simulink model "Continuos_plant_LTV_system"  (R2016b)
settings: Solver=ode3  StartTime=0.0  StopTime=1  FixedStep=0.01  RelTol=1e-6
libraries: dspinverses x1
settings Model: Creator=Utente  LastModifiedBy=liana
settings DataIOCC: SaveState=on
settings OptimizationCC: BlockReduction=off  DefaultParameterBehavior=Inlined  BufferReuse=off

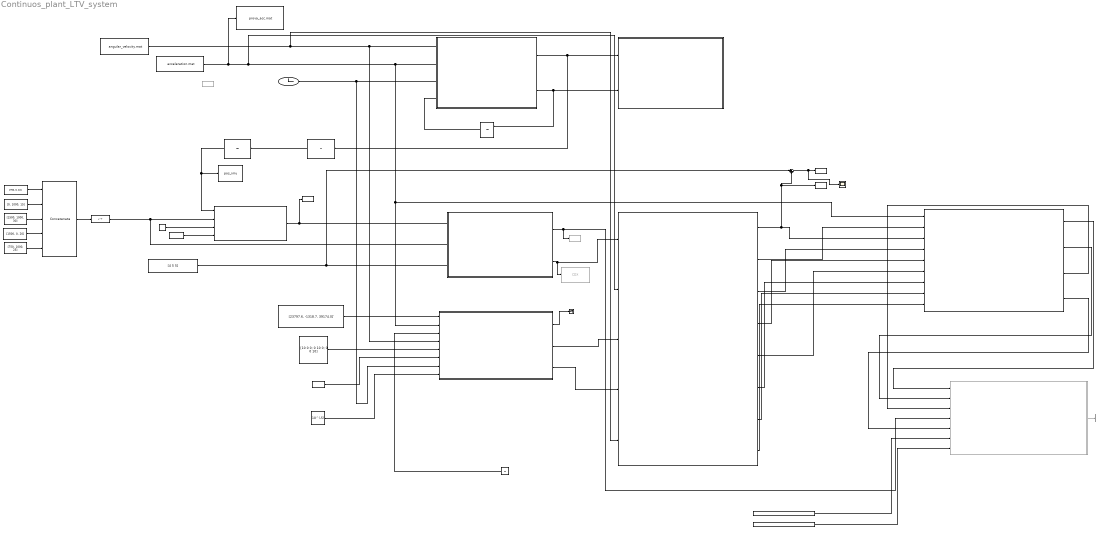
== system Continuos_plant_LTV_system ==
  Attitude Observer : Subsystem
  Clock : Clock
      settings: Decimation=50
  Displays : Subsystem
  From acceleration file : FromFile  FileName=acceleration.mat  SampleTime=0
  From angular_velocity file : FromFile  FileName=angular_velocity.mat  SampleTime=0
  Integrator : Integrator  InitialConditionSource=external
  Integrator1 : Integrator
  Integrator2 : Integrator
  Kalman - Bucy Filter : Subsystem  Commented=on
  Kp : Constant  Value=[10 0 0; 0 10 0; 0 0 10]
  Local linearization1 : Subsystem
  Math Function : Math  Operator=transpose  SaturateOnIntegerOverflow=on
  Matrix Concatenate (transponders positions) : Concatenate  NumInputs=5  Mode=Multidimensional array  ConcatenateDimension=2
  Mechanisation subsystem : Subsystem
  Nonlinear algebraic transform and solution : Subsystem
  Q matrix : Constant  Value=diag([0, 0, 0, 10^-5, 10^-3, 10^-3, 10^-3, 10^-8, 10^-8, 10^-8])
  R matrix : Constant  Value=0.25*diag([1 1 1 1])
  Scope : Scope
  Sum : Sum  Inputs=|++
  Terminator1 : Terminator
  Terminator2 : Terminator  Commented=on
  To File : ToFile  Filename=prova_acc.mat  MatrixName=prova_acc  SaveFormat=Timeseries
  To Workspace : ToWorkspace  VariableName=pseudo  SaveFormat=Timeseries  SampleTime=-1
  To Workspace1 : ToWorkspace  VariableName=pos_imu  SaveFormat=Timeseries  SampleTime=-1
  To Workspace2 : ToWorkspace  Commented=on  VariableName=CDX  SaveFormat=Timeseries  SampleTime=-1
  To Workspace3 : ToWorkspace  Commented=on  VariableName=acc_test  SaveFormat=Timeseries  SampleTime=-1
  To Workspace4 : ToWorkspace  VariableName=p_n  SaveFormat=Timeseries  SampleTime=-1
  To Workspace5 : ToWorkspace  VariableName=p_n_delta_stim  SaveFormat=Timeseries  SampleTime=-1
  To Workspace6 : ToWorkspace  Commented=on  VariableName=delta  SaveFormat=Timeseries  SampleTime=-1
  Translational Motion Observer : Subsystem
  Unit Delay : UnitDelay  SampleTime=-1
  beta : Constant
  epsilon : Constant  Value=[1 1 1 1 1]*0.1
  ki : Constant  Value=10^(-5)
  magneto_values (Pisa) : Constant  Value=[23797.6, -1318.7, 39174.0]'
  p_n_1 : Constant  Value=[750, 0, 10]
  p_n_2 : Constant  Value=[0, 1000, 15]
  p_n_3 : Constant  Value=[1500, 1000, 30]
  p_n_4 : Constant  Value=[1500, 0, 20]
  p_n_5 : Constant  Value=[750, 1000, 25]
  position_0_fixed_reference : Constant  Value=[4 5 5]
  pseudorange_measurement_model : MATLAB Function  TreatAsAtomicUnit=on
  sigma : Constant  Value=0.25
  wires:
  Clock/1 -> Attitude Observer/7(t), Mechanisation subsystem/3(t)
  Mechanisation subsystem/1(v_n_dot) -> Integrator1/1, Displays/1(v_n_dot)
  Mechanisation subsystem/2(R_nb_dot) -> Integrator/1, Displays/2(R_nb_dot)
  Nonlinear algebraic transform and solution/1(delta) -> To Workspace6/1, Kalman - Bucy Filter/4(sensors measurements)
  Kp/1 -> Attitude Observer/5(Kp)
  sigma/1 -> Attitude Observer/6(sigma)
  Nonlinear algebraic transform and solution/2(C_dx) -> Translational Motion Observer/1(C_dx_), To Workspace2/1
  Local linearization1/1(AL) -> Kalman - Bucy Filter/1(AL)
  Local linearization1/2(BL) -> Kalman - Bucy Filter/2(BL)
  Local linearization1/3(CL) -> Kalman - Bucy Filter/3(CL)
  pseudorange_measurement_model/1(y) -> To Workspace/1, Nonlinear algebraic transform and solution/1(y)
  Local linearization1/4(U) -> Kalman - Bucy Filter/5(U)
  beta/1 -> pseudorange_measurement_model/3(beta)
  epsilon/1 -> pseudorange_measurement_model/4(epsilon)
  Matrix Concatenate (transponders positions)/1 -> Math Function/1
  R matrix/1 -> Kalman - Bucy Filter/6(R)
  Q matrix/1 -> Kalman - Bucy Filter/7(Q)
  Kalman - Bucy Filter/1(Out1) -> Terminator2/1
  ki/1 -> Attitude Observer/8(Ki)
  Unit Delay/1 -> Attitude Observer/3(f_n_stim)
  p_n_5/1 -> Matrix Concatenate (transponders positions)/5
  p_n_4/1 -> Matrix Concatenate (transponders positions)/4
  p_n_3/1 -> Matrix Concatenate (transponders positions)/3
  p_n_2/1 -> Matrix Concatenate (transponders positions)/2
  p_n_1/1 -> Matrix Concatenate (transponders positions)/1
  Math Function/1 -> Nonlinear algebraic transform and solution/2(p), pseudorange_measurement_model/2(p_n_i)
  From angular_velocity file/1 -> Translational Motion Observer/5(w_b_ib_), Attitude Observer/4(w_ib), Mechanisation subsystem/1(w_ib)
  From acceleration file/1 -> To File/1, Translational Motion Observer/2(f_b_), Local linearization1/1(f_b_imu), Attitude Observer/2(f_b), Mechanisation subsystem/2(f_b)
  Sum/1 -> Scope/1, To Workspace4/1
  position_0_fixed_reference/1 -> Sum/1, Nonlinear algebraic transform and solution/3(p0)
  Integrator/1 -> Mechanisation subsystem/4("R_nb ")
  Integrator2/1 -> To Workspace1/1, pseudorange_measurement_model/1(p_n)
  magneto_values (Pisa)/1 -> Attitude Observer/1(m_b_mag)
  Integrator1/1 -> Integrator2/1
  Translational Motion Observer/2(beta_stim_) -> Local linearization1/2(beta_stim)
  Translational Motion Observer/5(K_) -> Local linearization1/6(K)
  Translational Motion Observer/1(p_n_delta_stim_) -> Sum/2, To Workspace5/1, Local linearization1/3(p_n_delta_stim)
  Translational Motion Observer/3(v_n_stim_) -> Local linearization1/4(v_n_stim)
  Translational Motion Observer/4(f_n_stim_) -> Local linearization1/5(f_n_stim)
  Translational Motion Observer/6(C_) -> Local linearization1/7(C)
  Translational Motion Observer/7(A_) -> Local linearization1/8(A)
  Translational Motion Observer/8(B_1_) -> Local linearization1/9(B)
  Attitude Observer/2(R_nb_stim) -> Translational Motion Observer/3("R_nb_stim_ ")
  Attitude Observer/1(J) -> Terminator1/1
  Attitude Observer/3(b_stim) -> Translational Motion Observer/4(b_stim)

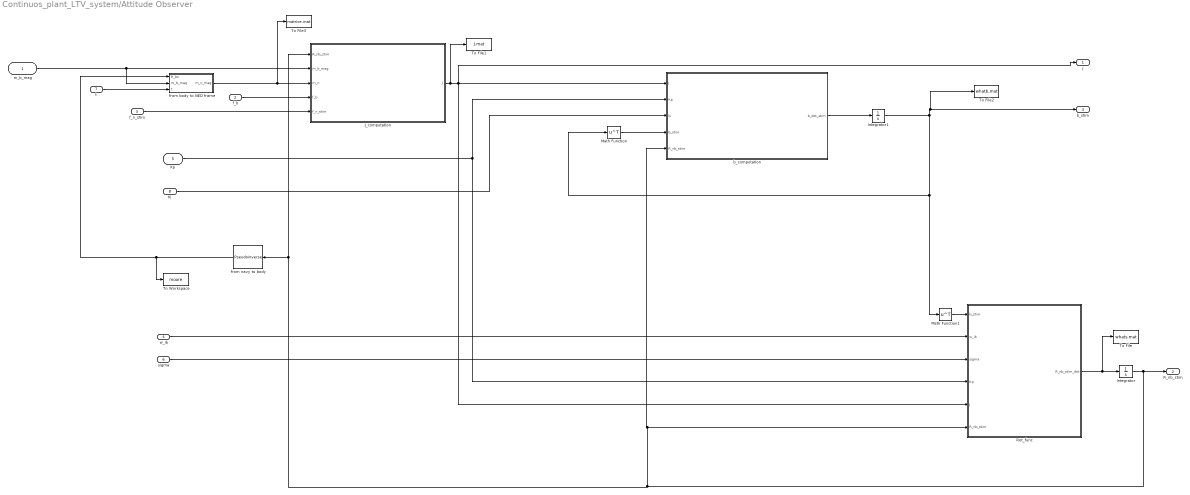
== system Continuos_plant_LTV_system/Attitude Observer ==
  m_b_mag : Inport
  f_b : Inport  Port=2
  f_n_stim : Inport  Port=3
  w_ib : Inport  Port=4
  Kp : Inport  Port=5
  sigma : Inport  Port=6
  t : Inport  Port=7
  Ki : Inport  Port=8
  Integrator : Integrator
  Integrator1 : Integrator
  J_computation : Subsystem
  Math Function : Math  Operator=transpose  SaturateOnIntegerOverflow=on
  Math Function1 : Math  Operator=transpose  SaturateOnIntegerOverflow=on
  Rot_func : MATLAB Function  TreatAsAtomicUnit=on
  To File : ToFile  Filename=whats.mat  MatrixName=ansm  SaveFormat=Timeseries
  To File1 : ToFile  Filename=J.mat  MatrixName=J  SaveFormat=Timeseries
  To File2 : ToFile  Filename=whatb.mat  MatrixName=b  SaveFormat=Timeseries
  To File3 : ToFile  Filename=matrice.mat  MatrixName=m  SaveFormat=Timeseries
  To Workspace : ToWorkspace  VariableName=moore  SaveFormat=Timeseries  SampleTime=-1
  b_computation : MATLAB Function  TreatAsAtomicUnit=on
  from body to NED frame : MATLAB Function  TreatAsAtomicUnit=on
  from navy to body : dspinverses/Pseudoinverse  wanterr=off  SimulateUsing=Interpreted execution
  J : Outport
  R_nb_stim : Outport  Port=2
  b_stim : Outport  Port=3
  wires:
  m_b_mag/1 -> from body to NED frame/2(m_b_mag), J_computation/2(m_b_mag)
  Rot_func/1(R_nb_stim_dot) -> Integrator/1, To File/1
  b_computation/1(b_dot_stim) -> Integrator1/1
  from body to NED frame/1(m_n_mag) -> To File3/1, J_computation/3(m_n)
  f_b/1 -> J_computation/4(f_b)
  f_n_stim/1 -> J_computation/5(f_n_stim)
  J_computation/1(J) -> To File1/1, J/1, Rot_func/5(J), b_computation/1(J)
  Kp/1 -> b_computation/2(Kp), Rot_func/4(Kp)
  Ki/1 -> b_computation/3(ki)
  sigma/1 -> Rot_func/3(sigma)
  w_ib/1 -> Rot_func/2(w_ib)
  t/1 -> from body to NED frame/3(t)
  Integrator1/1 -> Math Function/1, Math Function1/1, To File2/1, b_stim/1
  Integrator/1 -> from navy to body/1, J_computation/1(R_nb_stim), b_computation/5(R_nb_stim), Rot_func/6(R_nb_stim), R_nb_stim/1
  from navy to body/1 -> To Workspace/1, from body to NED frame/1(R_bn)
  Math Function/1 -> b_computation/4(b_stim)
  Math Function1/1 -> Rot_func/1(b_stim)

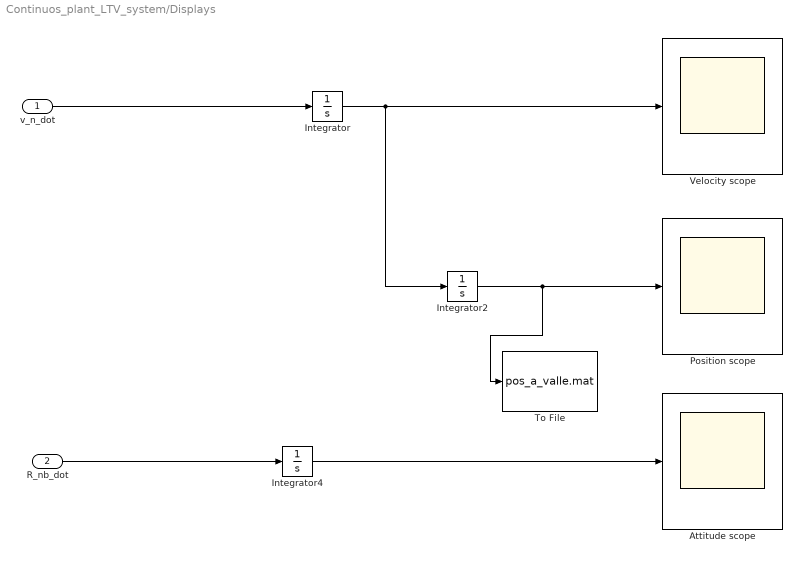
== system Continuos_plant_LTV_system/Displays ==
  v_n_dot : Inport
  R_nb_dot : Inport  Port=2
  Attitude scope : Scope
  Integrator : Integrator
  Integrator2 : Integrator
  Integrator4 : Integrator
  Position scope : Scope
  To File : ToFile  Filename=pos_a_valle.mat  MatrixName=pos_valle  SaveFormat=Timeseries
  Velocity scope : Scope
  wires:
  v_n_dot/1 -> Integrator/1
  Integrator/1 -> Integrator2/1, Velocity scope/1
  Integrator2/1 -> To File/1, Position scope/1
  R_nb_dot/1 -> Integrator4/1
  Integrator4/1 -> Attitude scope/1

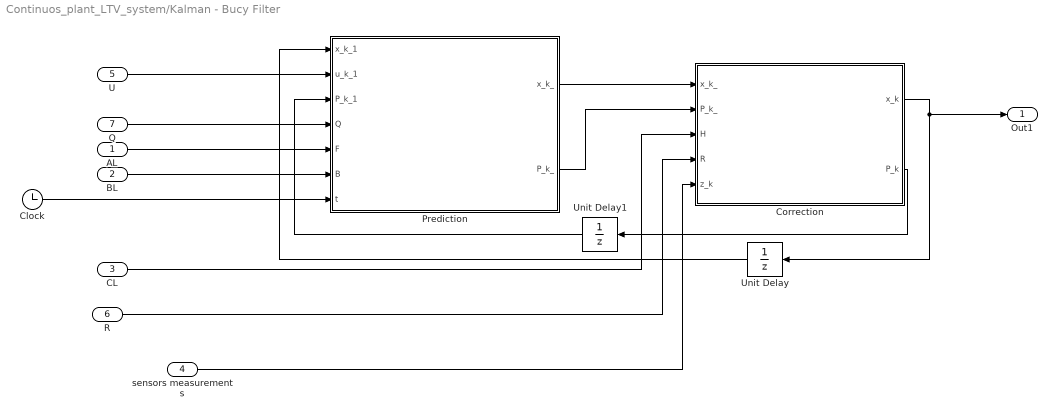
== system Continuos_plant_LTV_system/Kalman - Bucy Filter ==
  AL : Inport
  BL : Inport  Port=2
  CL : Inport  Port=3
  sensors measurements : Inport  Port=4
  U : Inport  Port=5
  R : Inport  Port=6
  Q : Inport  Port=7
  Clock : Clock
  Correction : MATLAB Function  TreatAsAtomicUnit=on
  Prediction : MATLAB Function  TreatAsAtomicUnit=on
  Unit Delay : UnitDelay  SampleTime=-1
  Unit Delay1 : UnitDelay  SampleTime=-1
  Out1 : Outport
  wires:
  Prediction/2(P_k_) -> Correction/2(P_k_)
  Prediction/1(x_k_) -> Correction/1(x_k_)
  Correction/2(P_k) -> Unit Delay1/1
  Correction/1(x_k) -> Unit Delay/1, Out1/1
  AL/1 -> Prediction/5(F)
  CL/1 -> Correction/3(H)
  Clock/1 -> Prediction/7(t)
  Q/1 -> Prediction/4(Q)
  sensors measurements/1 -> Correction/5(z_k)
  BL/1 -> Prediction/6(B)
  U/1 -> Prediction/2(u_k_1)
  R/1 -> Correction/4(R)
  Unit Delay/1 -> Prediction/1(x_k_1)
  Unit Delay1/1 -> Prediction/3(P_k_1)

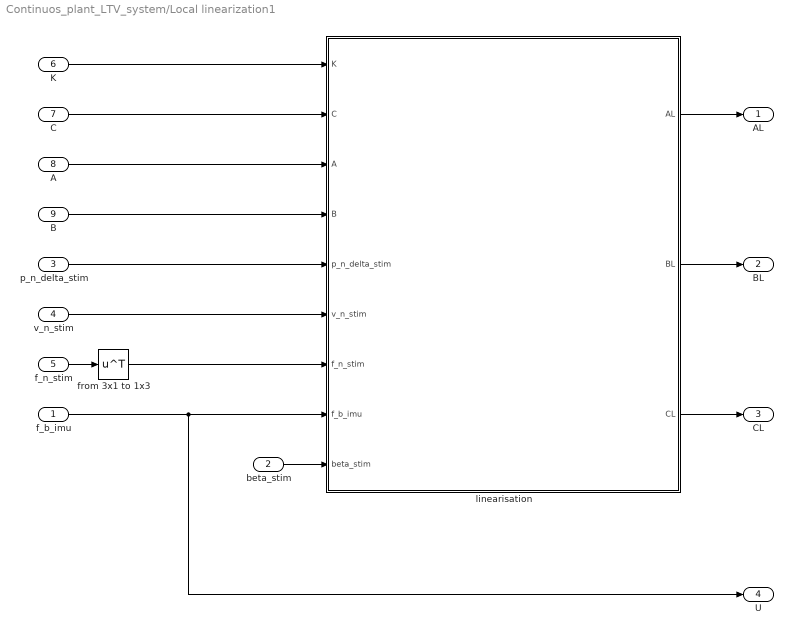
== system Continuos_plant_LTV_system/Local linearization1 ==
  f_b_imu : Inport
  beta_stim : Inport  Port=2
  p_n_delta_stim : Inport  Port=3
  v_n_stim : Inport  Port=4
  f_n_stim : Inport  Port=5
  K : Inport  Port=6
  C : Inport  Port=7
  A : Inport  Port=8
  B : Inport  Port=9
  from 3x1 to 1x3 : Math  Operator=transpose  SaturateOnIntegerOverflow=on
  linearisation : MATLAB Function  TreatAsAtomicUnit=on
  AL : Outport
  BL : Outport  Port=2
  CL : Outport  Port=3
  U : Outport  Port=4
  wires:
  linearisation/1(AL) -> AL/1
  linearisation/2(BL) -> BL/1
  linearisation/3(CL) -> CL/1
  K/1 -> linearisation/1(K)
  C/1 -> linearisation/2(C)
  A/1 -> linearisation/3(A)
  B/1 -> linearisation/4(B)
  p_n_delta_stim/1 -> linearisation/5(p_n_delta_stim)
  beta_stim/1 -> linearisation/9(beta_stim)
  f_n_stim/1 -> from 3x1 to 1x3/1
  v_n_stim/1 -> linearisation/6(v_n_stim)
  from 3x1 to 1x3/1 -> linearisation/7(f_n_stim)
  f_b_imu/1 -> U/1, linearisation/8(f_b_imu)

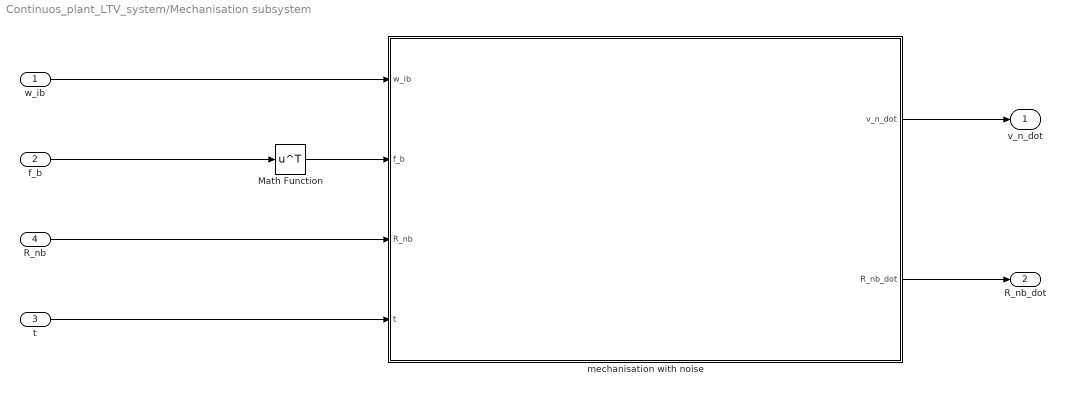
== system Continuos_plant_LTV_system/Mechanisation subsystem ==
  w_ib : Inport
  f_b : Inport  Port=2
  t : Inport  Port=3
  "R_nb " : Inport  Port=4
  Math Function : Math  Operator=transpose  SaturateOnIntegerOverflow=on
  mechanisation with noise : MATLAB Function  TreatAsAtomicUnit=on
  v_n_dot : Outport
  R_nb_dot : Outport  Port=2
  wires:
  w_ib/1 -> mechanisation with noise/1(w_ib)
  t/1 -> mechanisation with noise/4(t)
  f_b/1 -> Math Function/1
  mechanisation with noise/1(v_n_dot) -> v_n_dot/1
  mechanisation with noise/2(R_nb_dot) -> R_nb_dot/1
  "R_nb "/1 -> mechanisation with noise/3(R_nb)
  Math Function/1 -> mechanisation with noise/2(f_b)

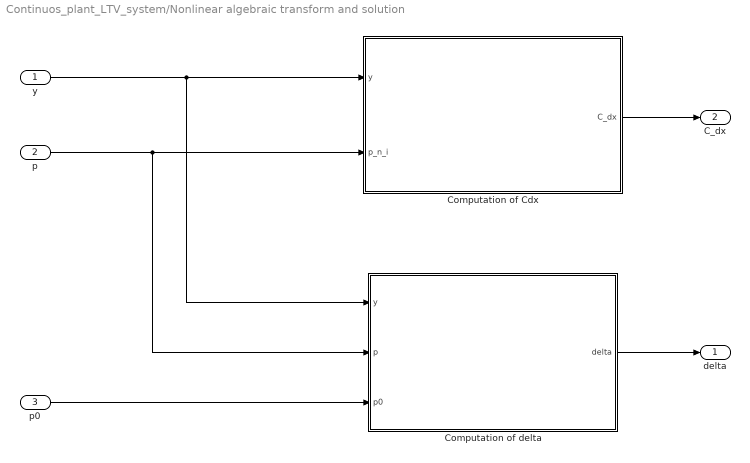
== system Continuos_plant_LTV_system/Nonlinear algebraic transform and solution ==
  y : Inport
  p : Inport  Port=2
  p0 : Inport  Port=3
  Computation of Cdx : MATLAB Function  TreatAsAtomicUnit=on
  Computation of delta : MATLAB Function  TreatAsAtomicUnit=on
  delta : Outport
  C_dx : Outport  Port=2
  wires:
  y/1 -> Computation of delta/1(y), Computation of Cdx/1(y)
  p/1 -> Computation of delta/2(p), Computation of Cdx/2(p_n_i)
  p0/1 -> Computation of delta/3(p0)
  Computation of delta/1(delta) -> delta/1
  Computation of Cdx/1(C_dx) -> C_dx/1

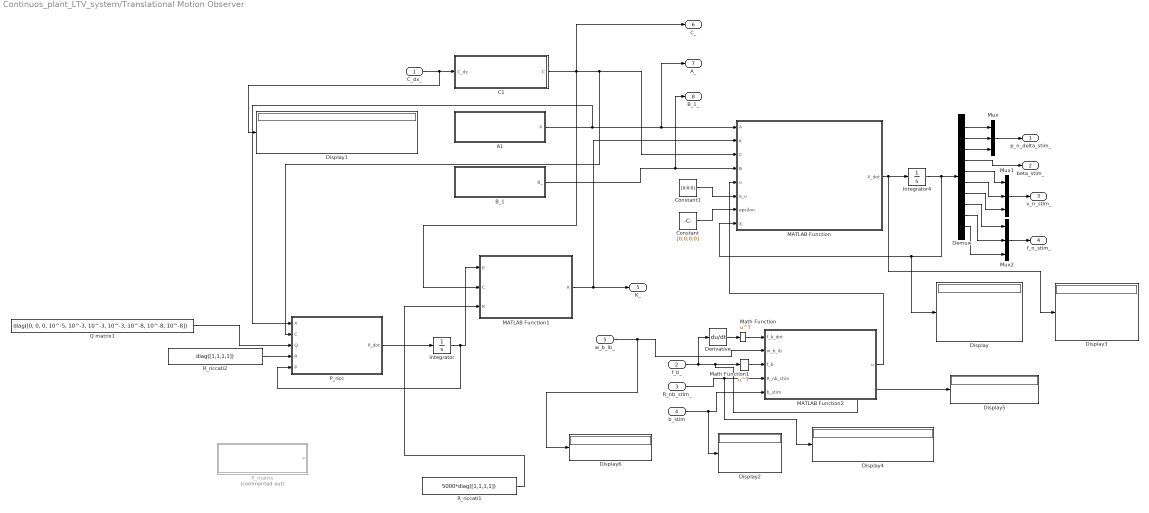
== system Continuos_plant_LTV_system/Translational Motion Observer ==
  C_dx_ : Inport
  f_b_ : Inport  Port=2
  "R_nb_stim_ " : Inport  Port=3
  b_stim : Inport  Port=4
  w_b_ib_ : Inport  Port=5
  A1 : MATLAB Function  TreatAsAtomicUnit=on
  B_1 : MATLAB Function  TreatAsAtomicUnit=on
  C1 : MATLAB Function  TreatAsAtomicUnit=on
  Constant : Constant  Value=[0;0;0;0]
  Constant1 : Constant  Value=[0;0;0]
  Demux : Demux  Outputs=10
  Derivative : Derivative
  Display{,1..6} (7 alike) : Display
  Integrator : Integrator
  Integrator4 : Integrator  AbsoluteTolerance=10^-9
  MATLAB Function : MATLAB Function  TreatAsAtomicUnit=on
  MATLAB Function1 : MATLAB Function  TreatAsAtomicUnit=on
  MATLAB Function2 : MATLAB Function  TreatAsAtomicUnit=on
  Math Function : Math  Operator=transpose  SaturateOnIntegerOverflow=on
  Math Function1 : Math  Operator=transpose  SaturateOnIntegerOverflow=on
  Mux : Mux  Inputs=3
  Mux1 : Mux  Inputs=3
  Mux2 : Mux  Inputs=3
  "P_matrix " : MATLAB Function  Commented=on  TreatAsAtomicUnit=on
  P_ricc : MATLAB Function  TreatAsAtomicUnit=on
  Q matrix1 : Constant  Value=diag([0, 0, 0, 10^-5, 10^-3, 10^-3, 10^-3, 10^-8, 10^-8, 10^-8])
  R_riccati1 : Constant  Value=5000*diag([1,1,1,1])
  R_riccati2 : Constant  Value=diag([1,1,1,1])
  p_n_delta_stim_ : Outport
  beta_stim_ : Outport  Port=2
  v_n_stim_ : Outport  Port=3
  f_n_stim_ : Outport  Port=4
  K_ : Outport  Port=5
  C_ : Outport  Port=6
  A_ : Outport  Port=7
  B_1_ : Outport  Port=8
  wires:
  MATLAB Function/1(X_dot) -> Display3/1, Integrator4/1
  Integrator4/1 -> Demux/1, Display/1, MATLAB Function/8(X)
  Demux/1 -> Mux/1
  Demux/2 -> Mux/2
  Demux/3 -> Mux/3
  Mux/1 -> p_n_delta_stim_/1
  Demux/4 -> beta_stim_/1
  Demux/5 -> Mux1/1
  Demux/6 -> Mux1/2
  Demux/7 -> Mux1/3
  Mux1/1 -> v_n_stim_/1
  Demux/8 -> Mux2/1
  Demux/9 -> Mux2/2
  Demux/10 -> Mux2/3
  Mux2/1 -> f_n_stim_/1
  A1/1(A) -> P_ricc/1(A), A_/1, MATLAB Function/1(A)
  C1/1(C) -> C_/1, MATLAB Function1/2(C), P_ricc/2(C), MATLAB Function/3(C)
  B_1/1(B_) -> B_1_/1, MATLAB Function/4(B)
  C_dx_/1 -> Display1/1, C1/1(C_dx)
  MATLAB Function1/1(K) -> K_/1, MATLAB Function/2(K)
  R_riccati1/1 -> MATLAB Function1/3(R)
  Constant/1 -> MATLAB Function/7(epsilon)
  MATLAB Function2/1(u) -> MATLAB Function/5(u)
  f_b_/1 -> Derivative/1, Display5/1, Math Function1/1
  "R_nb_stim_ "/1 -> Display4/1, MATLAB Function2/4(R_nb_stim)
  b_stim/1 -> Display2/1, MATLAB Function2/5(b_stim)
  w_b_ib_/1 -> Display6/1, MATLAB Function2/2(w_b_ib)
  Constant1/1 -> MATLAB Function/6(e_u)
  P_ricc/1(P_dot) -> Integrator/1
  Integrator/1 -> P_ricc/5(P), MATLAB Function1/1(P)
  R_riccati2/1 -> P_ricc/4(R)
  Q matrix1/1 -> P_ricc/3(Q)
  Derivative/1 -> Math Function/1
  Math Function/1 -> MATLAB Function2/1(f_b_dot)
  Math Function1/1 -> MATLAB Function2/3(f_b)

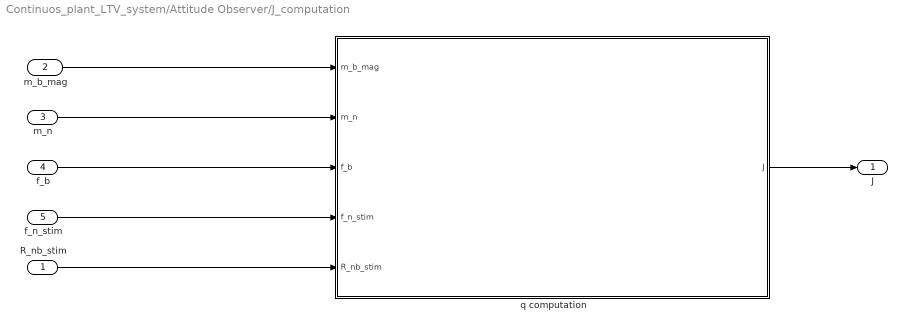
== system Continuos_plant_LTV_system/Attitude Observer/J_computation ==
  R_nb_stim : Inport
  m_b_mag : Inport  Port=2
  m_n : Inport  Port=3
  f_b : Inport  Port=4
  f_n_stim : Inport  Port=5
  q computation : MATLAB Function  TreatAsAtomicUnit=on
  J : Outport
  wires:
  m_n/1 -> q computation/2(m_n)
  f_n_stim/1 -> q computation/4(f_n_stim)
  m_b_mag/1 -> q computation/1(m_b_mag)
  f_b/1 -> q computation/3(f_b)
  q computation/1(J) -> J/1
  R_nb_stim/1 -> q computation/5(R_nb_stim)

== matlab function Continuos_plant_LTV_system/Translational Motion Observer/P_ricc ==
  data: P_dot output size=[10,10]; A input; C input; Q input; R input; P input
function P_dot = P(A, C, Q, R, P)

    P_dot = P*A + A'*P - P*C'*inv(R)*C*P + Q;
 
end

== matlab function Continuos_plant_LTV_system/Attitude Observer/J_computation/q computation ==
  data: m_b_mag input; m_n input; f_b input; f_n_stim input size=3; J output; R_nb_stim input size=[3,3]
function J  = qEfunc(m_b_mag, m_n, f_b, f_n_stim, R_nb_stim)

g_n = [0 0 9.81]';

q1_b = m_b_mag/norm(m_b_mag,2);
q2_b = f_b/norm(g_n,2);

q1_n = m_n/norm(m_n,2);
q2_n = f_n_stim/norm(g_n,2);


E_b = [q1_b, skew(q1_b)*q2_b', (skew(q1_b)*skew(q1_b))*q2_b'];
E_n = [q1_n, skew(q1_n)*q2_n, (skew(q1_n)*skew(q1_n))*q2_n];

J = (E_n - R_nb_stim * E_b) * (E_b');

end

== matlab function Continuos_plant_LTV_system/Kalman - Bucy Filter/Prediction ==
  data: x_k_1 input size=[10, 1]; x_k_ output; u_k_1 input; P_k_1 input size=[10,10]; Q input; F input; B input; P_k_ output; t input
function [x_k_, P_k_] = prediction(x_k_1, u_k_1, P_k_1, Q, F,B, t)

    % initial value of x_k_1
    if t == 0
        x_k_1 = zeros(10,1);
    end

    x_k_ = F * x_k_1 + B * u_k_1';
    
    P_k_ = F * P_k_1 * F' + Q;
    

end

== matlab function Continuos_plant_LTV_system/Mechanisation subsystem/mechanisation with noise ==
  data: w_ib input; f_b input; v_n_dot output; R_nb_dot output; R_nb input; t input
function [v_n_dot, R_nb_dot] = mechanisation(w_ib, f_b, R_nb, t)



g_n = [0 0 1]';

% w_ib = size(3,1);

if t == 0
    v_n_dot = zeros(3,1);
    R_nb_dot = eye(3);
    R_nb = eye(3);
end

Skew = skew(w_ib);


%p_dot = v_n;

v_n_dot = R_nb * f_b + g_n;

R_nb_dot = R_nb * Skew;

== matlab function Continuos_plant_LTV_system/Attitude Observer/b_computation ==
  data: J input; b_dot_stim output size=3; Kp input; ki input; b_stim input; R_nb_stim input
function b_dot_stim = b_dot_stim_func(J, Kp, ki, b_stim, R_nb_stim)

% don't break balls if there are too rows

%b_dot_stim = zeros(3 ,1);

% if t == 0
%    
%     b_stim = zeros(3, 1);
%     
% end

SAT = sat(R_nb_stim)';
PA = pa( SAT * Kp * J);
VEX = vexfunc(PA);
b_dot_stim = Proj(b_stim , -ki * VEX);

end

== matlab function Continuos_plant_LTV_system/Nonlinear algebraic transform and solution/Computation of Cdx ==
  data: y input; p_n_i input; C_dx output size=[4,4]
function C_dx  = C_dx_func(y,p_n_i)

    % y vector 
    % p matrix has row vectors
    %            (x,y,z) cols 
    %            m-rows are transponders number
    % all variables are in navigation frame oh yeah! baby ;)
    
    [row,col] = size(p_n_i);
    [row_,col_] = size(y);
    
    % m-measure vector
    p_m = p_n_i(row,:); % measure of m-th transponder
    y_m = y(row_);  % m-th pseudorange measure

    m = row; % m is transpoders number
    
    
    p_ = zeros(m-1,3); %row vector, 3 stands for x,y,z
    y_ = zeros(m-1,1);
    
    for i = 1 : 1 : m-1
    
        p_(i,:) = p_m - p_n_i(i,:);
        y_(i) = y(i) - y_m;
        
    end
    
    C_dx = [p_, y_];

end

== matlab function Continuos_plant_LTV_system/Nonlinear algebraic transform and solution/Computation of delta ==
  data: y input; delta output size=4; p input; p0 input
function delta  = delta_func(y, p, p0)

    % y vector 
    % p matrix has row vectors
    %            (x,y,z) cols 
    %            m-rows are the numbers of the transponders
    % all variables are in navigation frame oh yeah! baby ;)
    % z is a col vector of scalars
    
    % we must choose p0 (a block)
    
    [row,col] = size(p);
    %[row_,col_] = size(y);
    
    p_los = zeros(row,col);
    z = zeros(row,1);   % dim = m x 1
    
    %defining los vector
    for i = 1:1:row
       p_los(i,:) = p(i,:) - p0';       % dim = m x 3
    end
    
    % p_los = p_los';
    
    for i = 1:1:row
        z(i)= ((y(i)^2) - norm(p_los(i,:))^2); % dim = m x 1
    end
    
%     z = z';
%     
%     delta = zeros(row-1,1);
%     z_m = z(end);
%     
%     for i = 1:1:row-1
%         delta(i) =  (z(i) - z_m); %amm fenito
%     end

    delta = zeros(row-1,1); %dim = (m-1) x 1
    z_m = z(row,1);
    
    for i=1:1:(row-1)
        delta(i,1) = z(i,1) - z_m;
    end

end

== matlab function Continuos_plant_LTV_system/Attitude Observer/Rot_func ==
  data: b_stim input; R_nb_stim_dot output; w_ib input; sigma input; Kp input; J input; R_nb_stim input
function R_nb_stim_dot = rot_func(b_stim,w_ib,sigma,Kp,J,R_nb_stim) 

Skew = skew(w_ib - b_stim);

R_nb_stim_dot = R_nb_stim * Skew + sigma * Kp * J;

== matlab function Continuos_plant_LTV_system/Kalman - Bucy Filter/Correction ==
  data: x_k_ input; P_k_ input size=[10,10]; H input; R input; z_k input; x_k output; P_k output
function [x_k, P_k] = correction(x_k_ ,P_k_, H, R, z_k)

    n = size(P_k_);


    K_k = P_k_ * H' * pinv(H * P_k_ * H' + R);
    
    x_k = x_k_ + K_k * (z_k - H * x_k_);
    
    P_k = (eye(n) - K_k * H)*P_k_;

end

== matlab function Continuos_plant_LTV_system/pseudorange_measurement_model ==
  data: p_n input; y output size=5; p_n_i input; beta input; epsilon input
function y = pseudorange_mea_model(p_n, p_n_i, beta, epsilon)

  %  row-vector

  y = zeros(size(p_n_i,1),1);

  for i = 1: size(p_n_i,1)

      rho = norm(p_n - p_n_i(i,:)');  % eq. 7
      
      y(i) = rho + beta + epsilon(i); % eq. 8 

  end
      
end

== matlab function Continuos_plant_LTV_system/Local linearization1/linearisation ==
  data: K input size=[10,4]; AL output size=[10,10]; BL output size=[10,3]; CL output size=[4,10]; C input size=[4,10]; A input size=[10,10]; B input size=[10,3]; p_n_delta_stim input size=[1,3]; v_n_stim input size=[1,3]; f_n_stim input size=[1,3]; f_b_imu input size=[1,3]; beta_stim input size=1
function [AL, BL, CL] = linearisation(K,C,A,B, p_n_delta_stim, v_n_stim, f_n_stim, f_b_imu, beta_stim)

 % building state vector
 % xsi = [p_n_stim ; beta_stim; v_n_stim; f_n_tim];
%   xsi = zeros(10,1);
%   xsi(1:3,1) = p_n_delta_stim;
%   xsi(4,1) = beta_stim;
%   xsi(5:7,1) = v_n_stim;
%   xsi(8:10,1) = f_n_stim;
 % coder.extrinsic('ss');
 % sys = ss(A-K*C,B,C,0);
% % getting work point
%coder.extrinsic('trim');
%[X,U,Y,DX] = trim('sys', xsi);

% computing linearisation model
%coder.extrinsic('linmod');
%[AL, BL, CL, DL] = linmod('sys',X,U);

  
AL = zeros(10,10);
BL = zeros(10,3);
CL = zeros(size(C,1), 10);


coder.extrinsic('LinearizationFun');

[Al,Bl,Cl] = LinearizationFun(K,C,A,B);

p_n0 = p_n_delta_stim(1, 1);
p_n1 = p_n_delta_stim (1,2);
p_n2 = p_n_delta_stim(1,3);

v_n0 = v_n_stim(1, 1);
v_n1 = v_n_stim(1,2);
v_n2 = v_n_stim(1,3);

f_n0 = f_n_stim(1,1);
f_n1 = f_n_stim(1,2);
f_n2 = f_n_stim(1,3);

f_b0 = f_b_imu(1,1);
f_b1 = f_b_imu(1,2);
f_b2 = f_b_imu(1,3);


coder.extrinsic('eval');

AL_ = eval(Al);
BL_ = eval(Bl);
CL_ = eval(Cl);

% AL_ = feval('Al', p_n0, p_n1, p_n2,v_n0, v_n1, v_n2, f_n0, f_n1, f_n2, beta_stim);
% BL_ = feval('Bl', f_b0, f_b1, f_b2);
% CL_ = feval('Cl', p_n0, p_n1, p_n2,v_n0, v_n1, v_n2, f_n0, f_n1, f_n2, beta_stim);
% 

AL = AL_;
BL = BL_;
CL = CL_;


end

== matlab function Continuos_plant_LTV_system/Attitude Observer/from body to NED frame ==
  data: R_bn input; m_n_mag output; m_b_mag input; t input
function m_n_mag = b2n(R_bn, m_b_mag, t)

if t==0
    R_bn = eye(3);
end

m_n_mag = R_bn * m_b_mag;

== matlab function Continuos_plant_LTV_system/Translational Motion Observer/MATLAB Function ==
  data: A input; K input; C input; B input; u input; X_dot output; e_u input; epsilon input; X input size=[10,1]
function X_dot = system(A, K, C, B, u, e_u, epsilon, X) 

    X_dot = (A-K*C)*X + B*u + B*e_u + K*epsilon;
    
end

== matlab function Continuos_plant_LTV_system/Translational Motion Observer/A1 ==
  data: A output
function A = A()

 A = zeros(10);

 A(1:3,5:7) = eye(3);
 A(5:7,8:10) = eye(3);
 
end

== matlab function Continuos_plant_LTV_system/Translational Motion Observer/B_1 ==
  data: B_ output
function B_ = B()

 B_ = zeros(10,3);

 B_(8:10,1:3) = eye(3);
end

== matlab function Continuos_plant_LTV_system/Translational Motion Observer/C1 ==
  data: C output; C_dx input
function C = Cfunc(C_dx)

   row = size(C_dx,1); 

   C1 = zeros(row,6);

 C = [2*C_dx C1];
 
 
end

== matlab function Continuos_plant_LTV_system/Translational Motion Observer/MATLAB Function1 ==
  data: P input; K output; C input; R input
function K = K_fun(P,C,R)

    K = P*C'*inv(R);
    
end

== matlab function Continuos_plant_LTV_system/Translational Motion Observer/P_matrix  ==
  data: P output
function P = P()

 P = eye(10);
 
end

== matlab function Continuos_plant_LTV_system/Translational Motion Observer/MATLAB Function2 ==
  data: u output; f_b_dot input; w_b_ib input; f_b input; R_nb_stim input; b_stim input
function u = input_fun(f_b_dot, w_b_ib, f_b, R_nb_stim, b_stim)

    b_tilde = -b_stim;
    R_tilde = -R_nb_stim;
    u = R_tilde*f_b_dot + R_tilde*skew(w_b_ib)*f_b - R_nb_stim*skew(b_tilde)*f_b;
    
end
